simulink model "simulacion_circuito"  (R2023a)
settings: Solver=VariableStepAuto  StartTime=0.0  StopTime=1/F  RelTol=1e-3
undefined symbols (not defined in the file): F
libraries: spsSeriesRLCBranchLib x3, spsFourierLib x2, spsACVoltageSourceLib x1, spsCurrentMeasurementLib x1, spsGroundLib x1, spsMultimeterLib x1, sps_lib x1
settings Model: Creator=Juan Esteban  LastModifiedBy=Juan Esteban

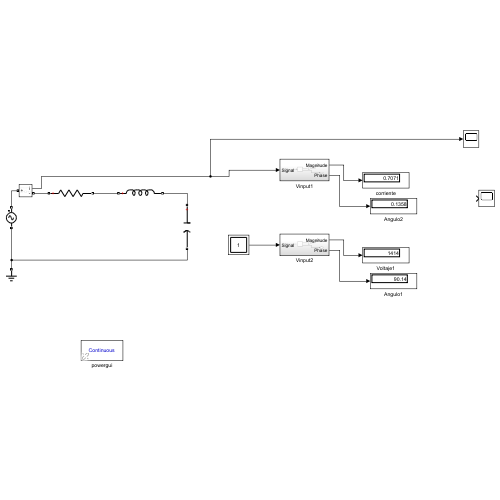
[thumbnail: Simulink's stored preview of the top-level diagram]
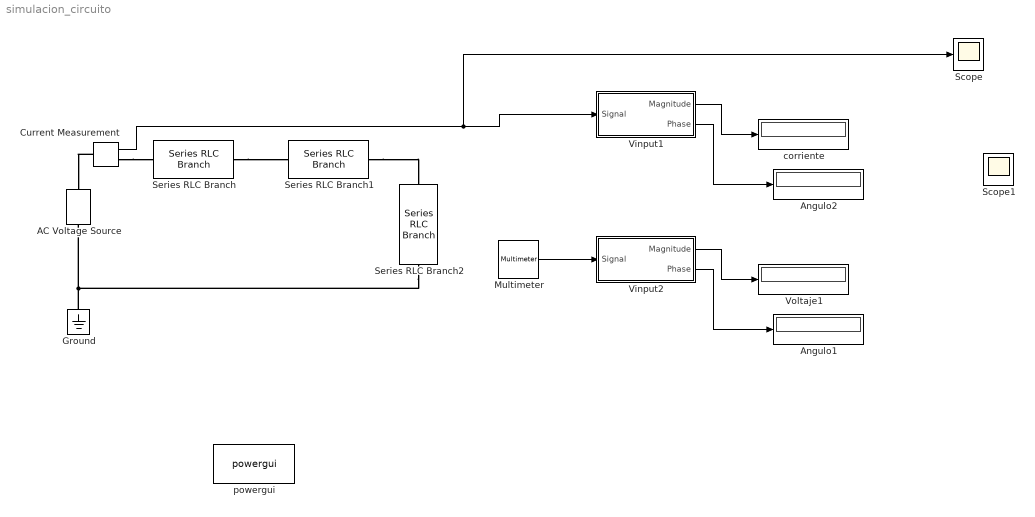
== system simulacion_circuito ==
  AC Voltage Source : spsACVoltageSourceLib/AC Voltage Source  Amplitude=10  Phase=0  Frequency=F  SampleTime=0  Measurements=None  BusType=swing  Pref=10e3  Qref=0  Qmin=-inf  Qmax=+inf
  Angulo1 : Display
  Angulo2 : Display
  Current Measurement : spsCurrentMeasurementLib/Current Measurement  PhasorSimulation=off  OutputType=Complex  PSBequivalent=0
  Ground : spsGroundLib/Ground  LConnTagsString=a
  Multimeter : spsMultimeterLib/Multimeter  L=1  sel=1  yselected={}  Gain=1  OutputType=Complex  PlotAtSimulationStop=off  PhasorSimulation=off
  Scope : Scope
  Scope1 : Scope
  Series RLC Branch : spsSeriesRLCBranchLib/Series RLC Branch  LConnTagsString=__new0  RConnTagsString=__new0  BranchType=R  Resistance=10  Inductance=1e-3  SetiL0=off  InitialCurrent=0  Capacitance=1e-6  Setx0=off  InitialVoltage=0  Measurements=None
  Series RLC Branch1 : spsSeriesRLCBranchLib/Series RLC Branch  LConnTagsString=__new0  RConnTagsString=__new0  BranchType=L  Resistance=1  Inductance=400e-3  SetiL0=off  InitialCurrent=0  Capacitance=1e-6  Setx0=off  InitialVoltage=0  Measurements=Branch voltage
  Series RLC Branch2 : spsSeriesRLCBranchLib/Series RLC Branch  LConnTagsString=__new0  RConnTagsString=__new0  BranchType=C  Resistance=1  Inductance=1e-3  SetiL0=off  InitialCurrent=0  Capacitance=100e-9  Setx0=off  InitialVoltage=0  Measurements=None
  Vinput1 : Subsystem
  Vinput2 : Subsystem
  Voltaje1 : Display
  corriente : Display
  powergui : sps_lib/powergui  Priority=1  SimulationMode=Continuous  SampleTime=50e-6  frequency=60  Iterations=50  frequencyindice=795.77  Pbase=100e6  ErrMax=1e-4  UnitsV=kV  UnitsW=MW  buscounter=0  FunctionMessages=off  echomessages=off  EnableUseOfTLC=off  CurrentSourceSwitches=off  DisableSnubberDevices=off  DisableRonSwitches=off  DisableVfSwitches=off  DisplayEquations=off  AutomaticDiscreteSolvers=off  SolverType=Tustin/Backward Euler (TBE)  Interpol=off  ExternalGateDelay=off  methode=off  Ts=100  x0status=blocks  SPID=on  SwTol=0  HookPort=off  NonlinearTolerance=1e-4  nMaxIteration=100  ContinueOnMaxIteration=off  RestoreLinks=warning  ResistiveCurrentMeasurement=off  Frange=[0:2:500]  Ylog=off  Xlog=on  ShowGrid=off  save=off  variable=ZData  structure=0  ZoomFFT=off  StartTime=0.0  cycles=1  DisplayStyle=1  fundamental=60  FreqAxis=off  MaxFrequency=1000  frequencyindicesteady=1  RmsSteady=1  display=off
  wires:
  Current Measurement/1 -> Scope/1, Vinput1/1(Signal)
  Vinput1/1(Magnitude) -> corriente/1
  Vinput1/2(Phase) -> Angulo2/1
  Vinput2/2(Phase) -> Angulo1/1
  Vinput2/1(Magnitude) -> Voltaje1/1
  Multimeter/1 -> Vinput2/1(Signal)
  connections:
  Series RLC Branch/RConn1 -- Series RLC Branch1/LConn1
  Series RLC Branch1/RConn1 -- Series RLC Branch2/LConn1
  Series RLC Branch2/RConn1 -- Ground/LConn1 -- AC Voltage Source/LConn1
  Current Measurement/LConn1 -- AC Voltage Source/RConn1
  Current Measurement/RConn1 -- Series RLC Branch/LConn1

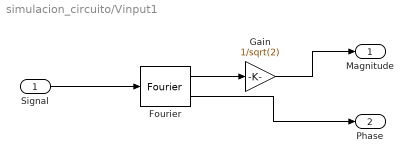
== system simulacion_circuito/Vinput1 ==
  Signal : Inport
  Fourier : spsFourierLib/Fourier  Freq=F  n=1  InInit=[0, 0]  Ts=0
  Gain : Gain  Gain=1/sqrt(2)
  Magnitude : Outport
  Phase : Outport  Port=2
  wires:
  Fourier/1 -> Gain/1
  Fourier/2 -> Phase/1
  Gain/1 -> Magnitude/1
  Signal/1 -> Fourier/1

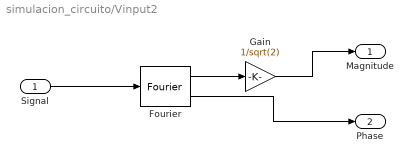
== system simulacion_circuito/Vinput2 ==
  Signal : Inport
  Fourier : spsFourierLib/Fourier  Freq=F  n=1  InInit=[0, 0]  Ts=0
  Gain : Gain  Gain=1/sqrt(2)
  Magnitude : Outport
  Phase : Outport  Port=2
  wires:
  Fourier/1 -> Gain/1
  Fourier/2 -> Phase/1
  Gain/1 -> Magnitude/1
  Signal/1 -> Fourier/1
